simulink model "L03"  (R2021a)
settings: Solver=FixedStepDiscrete  StartTime=0.0  StopTime=60.0  FixedStep=0.01  RelTol=1e-3
values from neighbouring files (symbols this model uses):
  Toff = 100    [Parameters.m]
  Ton = 200    [Parameters.m]
undefined symbols (not defined in the file or in its folder): sigbuilder_block
settings Model: Creator=ncleju  LastModifiedBy=ncleju

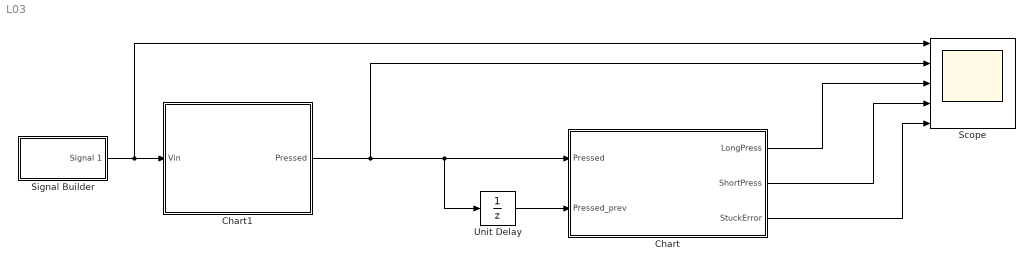
== system L03 ==
  Chart : Stateflow chart  TreatAsAtomicUnit=on
  Chart1 : Stateflow chart  TreatAsAtomicUnit=on
  Scope : Scope  NumInputPorts=5
  Signal Builder : Subsystem  Tag=STV Subsys  LoadFcn=sigbuilder_block('load');  StartFcn=sigbuilder_block('start');  StopFcn=sigbuilder_block('stop');  ClipboardFcn=sigbuilder_block('clipboard');  mask(Sigbuilder block){tuvar=[0:10]}
      mask help: Simulink:masks:SigbuilderBlock_MD
      mask init:
      | if ~strcmp(get_param(bdroot(gcbh),'SimulationStatus'),'stopped') tuvar = sigbuilder_block('maskInit'); end
      settings: CopyFcn=sigbuilder_block('copy');  DeleteFcn=sigbuilder_block('delete');  ModelCloseFcn=sigbuilder_block('modelClose');  PreSaveFcn=sigbuilder_block('preSave');  PauseFcn=sigbuilder_block('pause');  ContinueFcn=sigbuilder_block('continue');  NameChangeFcn=sigbuilder_block('namechange');  OpenFcn=sigbuilder_block('open',[6 30 1428 681.75 ]);  CloseFcn=sigbuilder_block('close');
      mask Display: plot(0, 0, 100, 100,[2, 2, 32, 32, 2], [68, 8, 8, 68, 68],[32, 2], [38, 38], [32, 19, 2],[53, 60, 44], [32, 17, 17, 2],[16, 16, 31, 31]);txt = getActiveGroup(gcbh);text(2, 100, txt,'verticalAlignment', 'top');
  Unit Delay : UnitDelay  SampleTime=-1  HasFrameUpgradeWarning=on
  wires:
  Signal Builder/1(Signal 1) -> Scope/1, Chart1/1(Vin)
  Chart1/1(Pressed) -> Scope/2, Chart/1(Pressed), Unit Delay/1
  Chart/1(LongPress) -> Scope/3
  Chart/2(ShortPress) -> Scope/4
  Unit Delay/1 -> Chart/2(Pressed_prev)
  Chart/3(StuckError) -> Scope/5

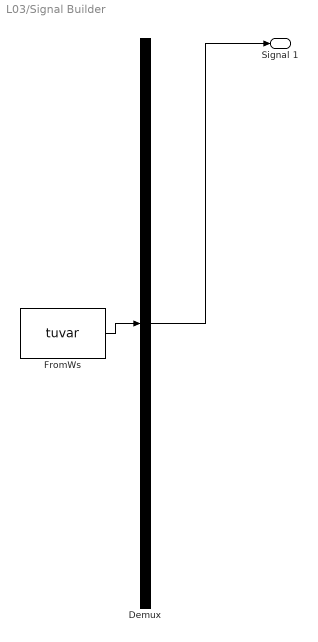
== system L03/Signal Builder ==
  Demux : Demux  Tag=STV Demux  Outputs=1
      settings: DisplayOption=none
  FromWs : FromWorkspace  Tag=STV FromWs  VariableName=tuvar
      SigBuilderData=|
      | common.afterFinalStr = 'Extrapolate'
      | common.sampleTime = 0
      | dataSet.timeRange = [0 60]
      | dataSet.name = 'Group 1'
      | sbobj.Groups.Name = 'Group 1'
      | sbobj.Groups.Signals.Name = 'Signal 1'
      | sbobj.Groups.Signals.XData = [0 1 1 1.15 1.19 2 2.1 2.5 2.6 2.65 2.66 3.56 3.57 3.95 4.13 45 45 49.55 50.15 52 53.3 60]
      | sbobj.Groups.Signals.YData = [5 4.62 0.18 0.22 4.7 4.66 0.33 0.38 5.1 5.02 0.2 0.24 4.69 4.67 0.14 0.17 4.74 4.76426666667 0.15 0.13 4.78426666667 4.82]
      | sbobj.Groups.TimeRange = [0 60]
  Signal 1 : Outport  Tag=STV Outport
  wires:
  Demux/1 -> Signal 1/1
  FromWs/1 -> Demux/1

== stateflow chart L03/Chart1 ==
  state NOTPRESSED
    en:
    Pressed=false;
  state WAIT2
  state WAIT1
  state PRESSED
    en:
    Pressed=true;
  (default) -> NOTPRESSED
  WAIT2 -> NOTPRESSED [order 1] : [after(Toff, msec)]
  NOTPRESSED -> WAIT1 : [Vin < 0.5]
  WAIT1 -> NOTPRESSED [order 2] : [Vin >= 0.5]
  WAIT1 -> PRESSED [order 1] : [after(Ton, msec)]
  PRESSED -> WAIT2 : [Vin > 4.5]
  WAIT2 -> PRESSED [order 2] : [Vin<=4.5]
  data: Vin input; Pressed output; Toff parameter; Ton parameter

== stateflow chart L03/Chart ==
  state IDLE
    en:
    ShortPress = false;
    StuckError = false;
  state SHORTPRESS
    en:
    ShortPress = true;
  state LETSWAIT
  state LONGPRESS
    en:
    LongPress = true;
  state CHECKERROR
    en:
    LongPress = false;
  state ERROR
    en:
    StuckError = true;
  ERROR -> IDLE : [Pressed == false]
  CHECKERROR -> IDLE [order 1] : [Pressed == false]
  (default) -> IDLE
  SHORTPRESS -> IDLE : [after(20, msec)]
  IDLE -> LETSWAIT : [Pressed == true]
  LETSWAIT -> SHORTPRESS [order 1] : [Pressed == false]
  LETSWAIT -> LONGPRESS [order 2] : [after(3000, msec)]
  LONGPRESS -> CHECKERROR : [after(20, msec)]
  CHECKERROR -> ERROR [order 2] : [after(21980, msec)]
  data: Pressed input; LongPress output; ShortPress output; Pressed_prev input; StuckError output
